simulink model "TWOAREAF"  (R2024b)
settings: Solver=VariableStepAuto  StartTime=0.0  StopTime=10.0  RelTol=1e-3
libraries: spspowerguiLib x1
settings Model: Creator=ADMIN  LastModifiedBy=ADMIN

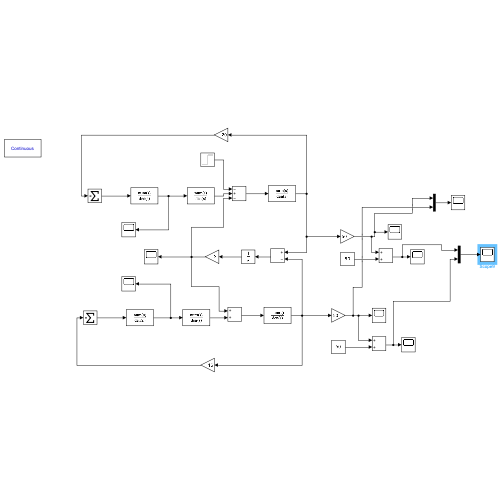
[thumbnail: Simulink's stored preview of the top-level diagram]
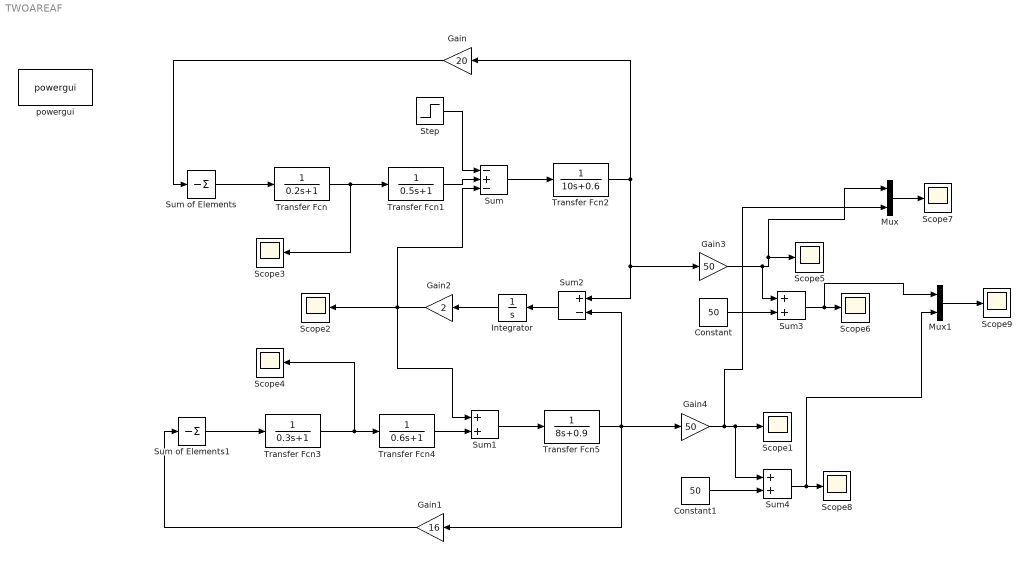
== system TWOAREAF ==
  Constant : Constant  Value=50
  Constant1 : Constant  Value=50
  Gain : Gain  Gain=20
  Gain1 : Gain  Gain=16
  Gain2 : Gain  Gain=2
  Gain3 : Gain  Gain=50
  Gain4 : Gain  Gain=50
  Integrator : Integrator
  Mux : Mux  Inputs=2
  Mux1 : Mux  Inputs=2
  Scope{1..9} (9 alike) : Scope
  Step : Step  Time=0  After=0.1875  SampleTime=0
  Sum : Sum  Inputs=-+-
  Sum of Elements : Sum  Inputs=-
  Sum of Elements1 : Sum  Inputs=-
  Sum1 : Sum
  Sum2 : Sum  Inputs=+-
  Sum3 : Sum
  Sum4 : Sum
  Transfer Fcn : TransferFcn  Denominator=[0.2 1]
  Transfer Fcn1 : TransferFcn  Denominator=[0.5 1]
  Transfer Fcn2 : TransferFcn  Denominator=[10 0.6]
  Transfer Fcn3 : TransferFcn  Denominator=[0.3 1]
  Transfer Fcn4 : TransferFcn  Denominator=[0.6 1]
  Transfer Fcn5 : TransferFcn  Denominator=[8 0.9]
  powergui : spspowerguiLib/powergui  Priority=1  SimulationMode=Continuous  SampleTime=50e-6  frequency=60  Iterations=50  frequencyindice=60  Pbase=100e6  ErrMax=1e-4  UnitsV=kV  UnitsW=MW  buscounter=0  FunctionMessages=off  echomessages=off  EnableUseOfTLC=off  CurrentSourceSwitches=off  DisableSnubberDevices=off  DisableRonSwitches=off  DisableVfSwitches=off  DisplayEquations=off  AutomaticDiscreteSolvers=off  SolverType=Tustin/Backward Euler (TBE)  Interpol=off  ExternalGateDelay=off  methode=off  Ts=100  x0status=blocks  SPID=on  SwTol=0  HookPort=off  NonlinearTolerance=1e-4  nMaxIteration=100  ContinueOnMaxIteration=off  RestoreLinks=warning  ResistiveCurrentMeasurement=off  Frange=[0:2:500]  Ylog=off  Xlog=on  ShowGrid=off  save=off  variable=ZData  structure=0  ZoomFFT=off  StartTime=0.0  cycles=1  DisplayStyle=1  fundamental=60  FreqAxis=off  MaxFrequency=1000  frequencyindicesteady=1  RmsSteady=1  display=off
  wires:
  Transfer Fcn/1 -> Scope3/1, Transfer Fcn1/1
  Transfer Fcn2/1 -> Gain3/1, Sum2/1, Gain/1
  Transfer Fcn1/1 -> Sum/2
  Step/1 -> Sum/1
  Gain/1 -> Sum of Elements/1
  Sum/1 -> Transfer Fcn2/1
  Sum of Elements/1 -> Transfer Fcn/1
  Gain1/1 -> Sum of Elements1/1
  Sum1/1 -> Transfer Fcn5/1
  Transfer Fcn4/1 -> Sum1/2
  Transfer Fcn3/1 -> Scope4/1, Transfer Fcn4/1
  Transfer Fcn5/1 -> Sum2/2, Gain4/1, Gain1/1
  Sum of Elements1/1 -> Transfer Fcn3/1
  Sum2/1 -> Integrator/1
  Integrator/1 -> Gain2/1
  Gain2/1 -> Sum1/1, Sum/3, Scope2/1
  Gain3/1 -> Sum3/1, Mux/1, Scope5/1
  Constant/1 -> Sum3/2
  Sum3/1 -> Mux1/1, Scope6/1
  Gain4/1 -> Mux/2, Sum4/1, Scope1/1
  Mux/1 -> Scope7/1
  Constant1/1 -> Sum4/2
  Sum4/1 -> Mux1/2, Scope8/1
  Mux1/1 -> Scope9/1
